simulink library "CrossProd"  (R2014b)
settings: Solver=VariableStepAuto  StartTime=0.0  StopTime=10.0  RelTol=1e-3
settings Model: Creator=y.akisheva  LastModifiedBy=Hp
settings DataIOCC: SaveFormat=Dataset
settings OptimizationCC: UseDivisionForNetSlopeComputation=off  SimCompilerOptimization=off
settings DebuggingCC: SolverPrmCheckMsg=none  FrameProcessingCompatibilityMsg=error  AllowSymbolicDim=off
settings HardwareCC: ProdBitPerPointer=64  ProdLargestAtomicFloat=Float  ProdIntDivRoundTo=Zero  ProdEndianess=LittleEndian  ProdWordSize=64  ProdHWDeviceType=Intel->x86-64 (Windows64)
settings RTWCC: RTWCompilerOptimization=off
settings GRTTargetCC: GeneratePreprocessorConditionals=Use local settings
settings ConfigComp: CovMetricSettings=dw  CovHtmlReporting=on  CovSaveCumulativeToWorkspaceVar=on  CovSaveSingleToWorkspaceVar=on  CovExternalEMLEnable=off

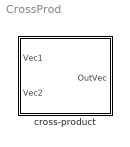
== system CrossProd ==
  cross-product : Subsystem

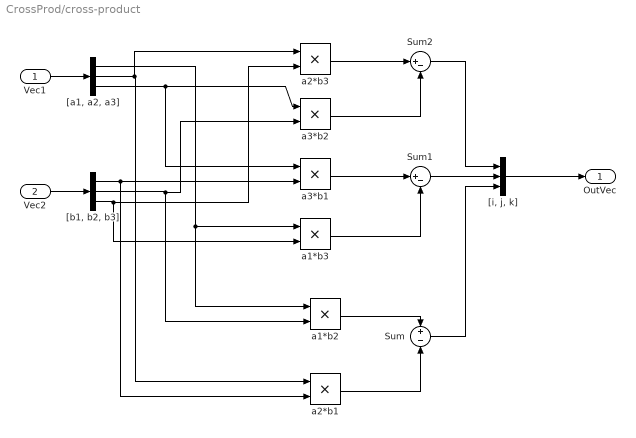
== system CrossProd/cross-product ==
  Vec1 : Inport
  Vec2 : Inport  Port=2
  Sum : Sum  Inputs=+-
  Sum1 : Sum  Inputs=|+-
  Sum2 : Sum  Inputs=|+-
  "[a1, a2, a3]" : Demux  Outputs=3
  "[b1, b2, b3]" : Demux  Outputs=3
  "[i, j, k]" : Mux  Inputs=3
  a1*b2 : Product
  a1*b3 : Product
  a2*b1 : Product
  a2*b3 : Product
  a3*b1 : Product
  a3*b2 : Product
  OutVec : Outport
  wires:
  Sum1/1 -> "[i, j, k]"/2
  Sum2/1 -> "[i, j, k]"/1
  Sum/1 -> "[i, j, k]"/3
  a3*b2/1 -> Sum2/2
  "[i, j, k]"/1 -> OutVec/1
  a1*b3/1 -> Sum1/2
  "[b1, b2, b3]"/3 -> a1*b3/2, a2*b3/2
  a2*b3/1 -> Sum2/1
  "[a1, a2, a3]"/3 -> a3*b2/1, a3*b1/1
  a3*b1/1 -> Sum1/1
  a1*b2/1 -> Sum/1
  "[b1, b2, b3]"/2 -> a1*b2/2, a3*b2/2
  Vec1/1 -> "[a1, a2, a3]"/1
  "[a1, a2, a3]"/1 -> a1*b2/1, a1*b3/1
  Vec2/1 -> "[b1, b2, b3]"/1
  "[a1, a2, a3]"/2 -> a2*b1/1, a2*b3/1
  "[b1, b2, b3]"/1 -> a2*b1/2, a3*b1/2
  a2*b1/1 -> Sum/2
